simulink model "subtask1_22_110107589"  (R2022a)
settings: Solver=FixedStepDiscrete  StartTime=0.0  StopTime=(28+1)*8-1  RelTol=1e-3  EnableMultiTasking=on
libraries: simulink x1
settings Model: LastModifiedBy=gowrav -local
settings SolverCC: AutoInsertRateTranBlk=on
settings ModelReferenceCC: EnableRefExpFcnMdlSchedulingChecks=off
settings RTWCC: Description=Generic Real-Time Target

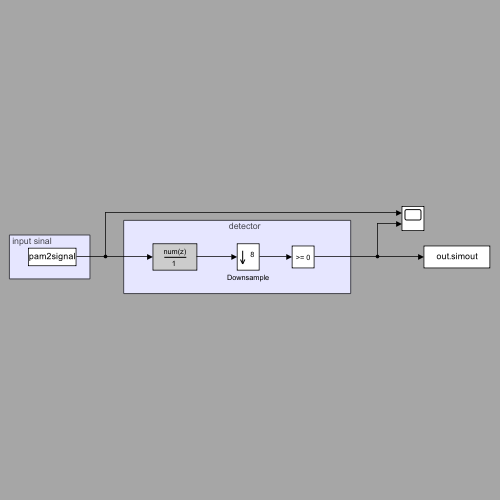
[thumbnail: Simulink's stored preview of the top-level diagram]
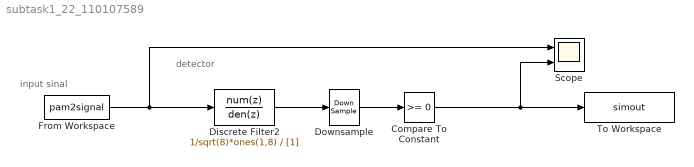
== system subtask1_22_110107589 ==
  note: input sinal
  note: detector
  Compare To Constant : simulink/Logic and Bit Operations/Compare To Constant  relop=>=  const=0  OutDataTypeStr=boolean
  Discrete Filter2 : DiscreteFilter  Numerator=1/sqrt(8)*ones(1,8)  Denominator=[1]
  Downsample : DownSample  N=8  phase=7  RateOptions=Allow multirate processing
  From Workspace : FromWorkspace  VariableName=pam2signal  SampleTime=1
  Scope : Scope  NumInputPorts=2
  To Workspace : ToWorkspace  VariableName=simout  SaveFormat=Timeseries  SampleTime=-1
  wires:
  Downsample/1 -> Compare To Constant/1
  Discrete Filter2/1 -> Downsample/1
  Compare To Constant/1 -> Scope/2, To Workspace/1
  From Workspace/1 -> Scope/1, Discrete Filter2/1
